simulink model "LEDS_BUENO"  (R2024b)
settings: Solver=VariableStepAuto  StartTime=0.0  StopTime=10.0  RelTol=1e-3
libraries: simulink x9, arduinolib x3
settings Model: Creator=Usuario  LastModifiedBy=Usuario

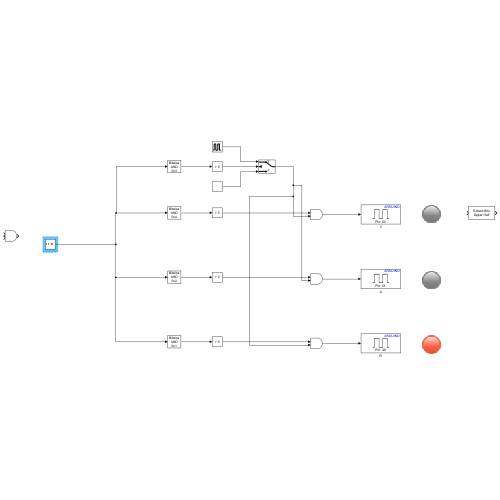
[thumbnail: Simulink's stored preview of the top-level diagram]
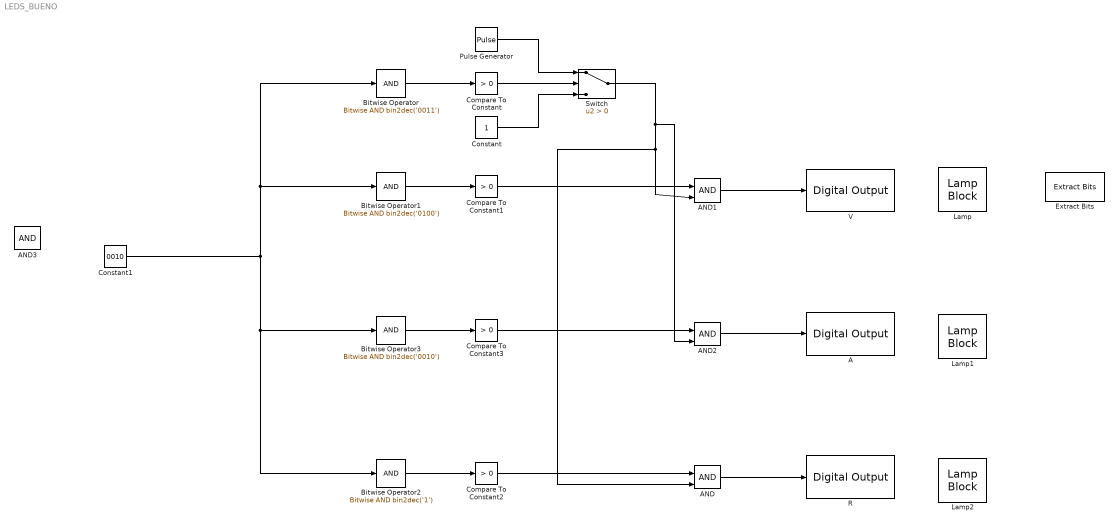
== system LEDS_BUENO ==
  A : arduinolib/Digital Output  pinNumber=51  Direction=output  blockPlatform=arduino
  AND{,1..3} (4 alike) : Logic  IconShape=distinctive  AllPortsSameDT=off  OutDataTypeStr=boolean
  Bitwise Operator : simulink/Logic and Bit Operations/Bitwise Operator  logicop=AND  UseBitMask=on  BitMask=bin2dec('0011')  BitMaskRealWorld=Stored Integer
  Bitwise Operator1 : simulink/Logic and Bit Operations/Bitwise Operator  logicop=AND  UseBitMask=on  BitMask=bin2dec('0100')  BitMaskRealWorld=Stored Integer
  Bitwise Operator2 : simulink/Logic and Bit Operations/Bitwise Operator  logicop=AND  UseBitMask=on  BitMask=bin2dec('1')  BitMaskRealWorld=Stored Integer
  Bitwise Operator3 : simulink/Logic and Bit Operations/Bitwise Operator  logicop=AND  UseBitMask=on  BitMask=bin2dec('0010')  BitMaskRealWorld=Stored Integer
  Compare To Constant{,1..3} (4 alike) : simulink/Logic and Bit Operations/Compare To Constant  relop=>  const=0  OutDataTypeStr=boolean
  Constant : Constant
  Constant1 : Constant  Value=0010  OutDataTypeStr=boolean
  Extract Bits : simulink/Logic and Bit Operations/Extract Bits  bitsToExtract=Upper half  numBits=8  bitIdxRange=[0 7]  outScalingMode=Preserve fixed-point scaling
  Lamp : LampBlock  LabelPosition=Hide
  Lamp1 : LampBlock  LabelPosition=Hide
  Lamp2 : LampBlock  LabelPosition=Hide
  Pulse Generator : DiscretePulseGenerator  PulseType=Time based  Period=10  PulseWidth=5
  R : arduinolib/Digital Output  pinNumber=49  Direction=output  blockPlatform=arduino
  Switch : Switch  Criteria=u2 > Threshold  SaturateOnIntegerOverflow=off  InputSameDT=off
  V : arduinolib/Digital Output  pinNumber=53  Direction=output  blockPlatform=arduino
  wires:
  AND2/1 -> A/1
  AND/1 -> R/1
  AND1/1 -> V/1
  Pulse Generator/1 -> Switch/1
  Switch/1 -> AND2/2, AND/2, AND1/2
  Compare To Constant/1 -> Switch/2
  Constant/1 -> Switch/3
  Bitwise Operator/1 -> Compare To Constant/1
  Compare To Constant1/1 -> AND1/1
  Bitwise Operator1/1 -> Compare To Constant1/1
  Bitwise Operator3/1 -> Compare To Constant3/1
  Compare To Constant3/1 -> AND2/1
  Bitwise Operator2/1 -> Compare To Constant2/1
  Compare To Constant2/1 -> AND/1
  Constant1/1 -> Bitwise Operator2/1, Bitwise Operator3/1, Bitwise Operator/1, Bitwise Operator1/1
